simulink subsystem "Staircase_Speed"  (R2022b)
settings: Solver=VariableStepAuto  StartTime=0.0  StopTime=10.0  RelTol=1e-3
libraries: simulink x1
settings Model: Creator=gotta  LastModifiedBy=gotta

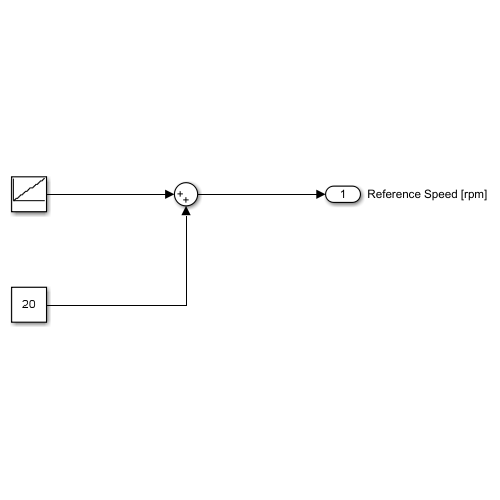
[thumbnail: Simulink's stored preview of the top-level diagram]
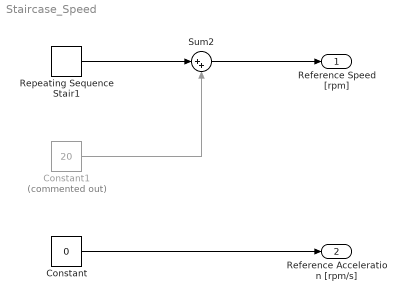
== system Staircase_Speed ==
  Constant : Constant  Value=0
  Constant1 : Constant  Commented=on  Value=20
  Repeating Sequence Stair1 : simulink/Sources/Repeating Sequence Stair  OutValues=5*[0:1:20]  tsamp=10  OutMin=[]  OutMax=[]  OutDataTypeStr=double  OutputDataTypeScalingMode=double  OutDataType=fixdt(0,8)  ConRadixGroup=Best Precision: Vector-wise  OutScaling=2^-12
  Sum2 : Sum  Inputs=|++
  Reference Speed [rpm] : Outport
  Reference Acceleration [rpm/s] : Outport  Port=2
  wires:
  Repeating Sequence Stair1/1 -> Sum2/1
  Constant1/1 -> Sum2/2
  Sum2/1 -> Reference Speed [rpm]/1
  Constant/1 -> Reference Acceleration [rpm/s]/1
